simulink library "csci_gsse_lib"  (R2014b)
settings: Solver=ode45  StartTime=0.0  StopTime=10.0  RelTol=1e-3
libraries: util_common_lib x2, util_info_lib x1, csc_gnd_sta_lib x1, csc_sim_simulation_lib x1, csc_valvesim_collection_lib x1, csu_cfe_cfe_time_lib x1, csu_tlm_telemetry_lib x1, csu_mems_mcu_signal_interface_lib x1, csu_tracker_mcu_signal_interface_lib x1, csu_valvesim_signal_interface_lib x1
settings Model: Creator=Mark Agbayani  LastModifiedBy=Mark Agbayani

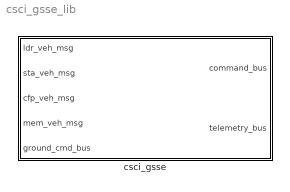
== system csci_gsse_lib ==
  csci_gsse : Subsystem

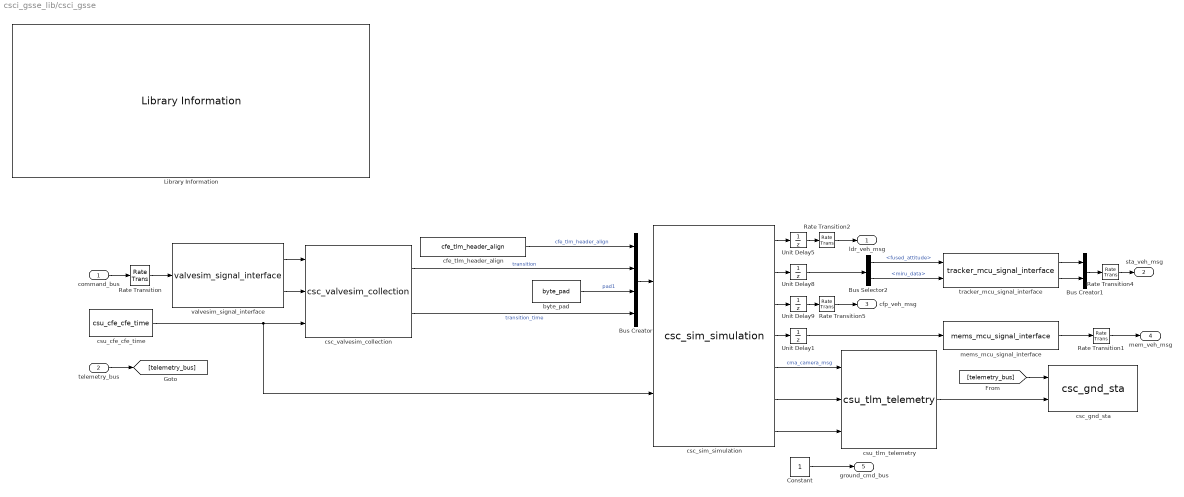
== system csci_gsse_lib/csci_gsse ==
  command_bus : Inport
  telemetry_bus : Inport  Port=2
  Bus Creator : BusCreator  OutDataTypeStr=Bus: thr_sim_msg  NonVirtualBus=on
  Bus Selector2 : BusSelector  OutputSignals=fused_attitude,miru_data
  Bus Creator1 : BusCreator  Inputs=2
  Constant : Constant
  Library Information : util_info_lib/Library Information  owner='NONE'
  Rate Transition{,1..2,4..5} (5 alike) : RateTransition  Integrity=off
  Unit Delay{1,5,8..9} (4 alike) : UnitDelay  SampleTime=-1
  byte_pad : util_common_lib/byte_pad  n_bytes=2
  cfe_tlm_header_align : util_common_lib/cfe_tlm_header_align
  csc_gnd_sta : csc_gnd_sta_lib/csc_gnd_sta  dir_name=scenario_data_dir
  csc_sim_simulation : csc_sim_simulation_lib/csc_sim_simulation  Tag=GSSE; MDL_TICK=THR_SIM_MSG
  csc_valvesim_collection : csc_valvesim_collection_lib/csc_valvesim_collection  SystemSampleTime=-1
  csu_cfe_cfe_time : csu_cfe_cfe_time_lib/csu_cfe_cfe_time  sch_dt=sim_time_step_size
  csu_tlm_telemetry : csu_tlm_telemetry_lib/csu_tlm_telemetry  num_inputs=3  output_bus_name=sim_telemetry_bus_msg
  mems_mcu_signal_interface : csu_mems_mcu_signal_interface_lib/mems_mcu_signal_interface
  tracker_mcu_signal_interface : csu_tracker_mcu_signal_interface_lib/tracker_mcu_signal_interface
  valvesim_signal_interface : csu_valvesim_signal_interface_lib/valvesim_signal_interface
  ldr_veh_msg : Outport
  sta_veh_msg : Outport  Port=2
  cfp_veh_msg : Outport  Port=3
  mem_veh_msg : Outport  Port=4
  ground_cmd_bus : Outport  Port=5
  wires:
  Rate Transition1/1 -> mem_veh_msg/1
  mems_mcu_signal_interface/1 -> Rate Transition1/1
  Unit Delay1/1 -> mems_mcu_signal_interface/1
  csc_sim_simulation/4 -> Unit Delay1/1
  Rate Transition4/1 -> sta_veh_msg/1
  Bus Creator1/1 -> Rate Transition4/1
  tracker_mcu_signal_interface/2 -> Bus Creator1/2
  tracker_mcu_signal_interface/1 -> Bus Creator1/1
  Unit Delay8/1 -> Bus Selector2/1
  Bus Selector2/2 -> tracker_mcu_signal_interface/2  "<miru_data>"
  Bus Selector2/1 -> tracker_mcu_signal_interface/1  "<fused_attitude>"
  valvesim_signal_interface/2 -> csc_valvesim_collection/2
  cfe_tlm_header_align/1 -> Bus Creator/1  "cfe_tlm_header_align"
  byte_pad/1 -> Bus Creator/3  "pad1"
  Bus Creator/1 -> csc_sim_simulation/1
  csc_valvesim_collection/2 -> Bus Creator/4  "transition_time"
  csc_valvesim_collection/1 -> Bus Creator/2  "transition"
  valvesim_signal_interface/1 -> csc_valvesim_collection/1
  Rate Transition/1 -> valvesim_signal_interface/1
  [telemetry_bus] -> csc_gnd_sta/1
  csu_tlm_telemetry/1 -> csc_gnd_sta/2
  csc_sim_simulation/7 -> csu_tlm_telemetry/3
  csc_sim_simulation/5 -> csu_tlm_telemetry/1  "cma_camera_msg"
  csc_sim_simulation/2 -> Unit Delay8/1
  Rate Transition5/1 -> cfp_veh_msg/1
  Rate Transition2/1 -> ldr_veh_msg/1
  command_bus/1 -> Rate Transition/1
  Constant/1 -> ground_cmd_bus/1
  csc_sim_simulation/3 -> Unit Delay9/1
  csc_sim_simulation/1 -> Unit Delay5/1
  Unit Delay5/1 -> Rate Transition2/1
  Unit Delay9/1 -> Rate Transition5/1
  csc_sim_simulation/6 -> csu_tlm_telemetry/2
  telemetry_bus/1 -> [telemetry_bus]
  csu_cfe_cfe_time/1 -> csc_sim_simulation/2, csc_valvesim_collection/3
